simulink model "assignment1_c"  (R2021a)
settings: Solver=VariableStepAuto  StartTime=0.0  StopTime=10.0  RelTol=1e-3
undefined symbols (not defined in the file): c1, c2, k1, k2, m1, m2
settings Model: Creator=mluser  LastModifiedBy=mluser

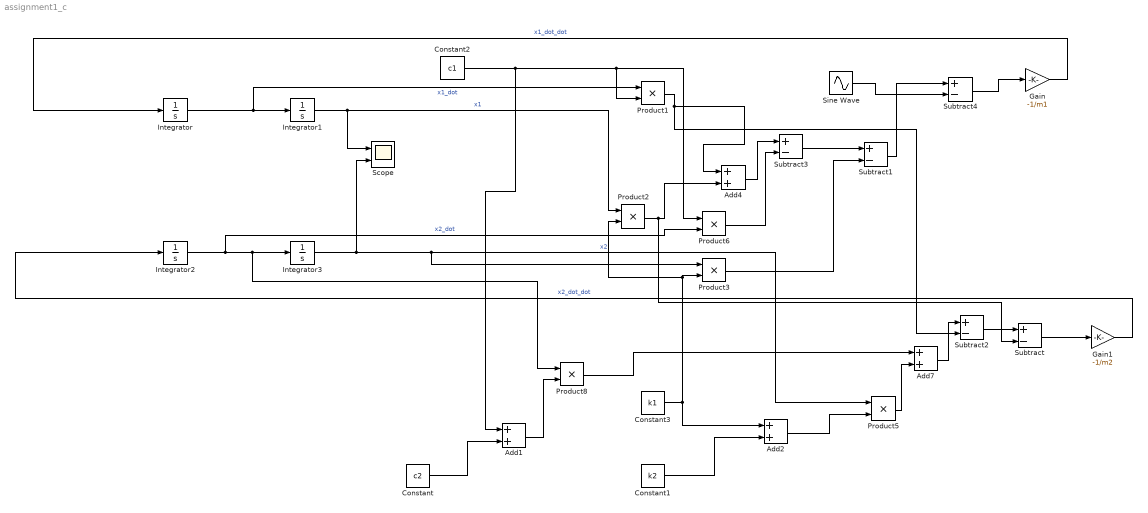
== system assignment1_c ==
  Add{1..2,4,7} (4 alike) : Sum
  Constant : Constant  Value=c2
  Constant1 : Constant  Value=k2
  Constant2 : Constant  Value=c1
  Constant3 : Constant  Value=k1
  Gain : Gain  Gain=-1/m1
  Gain1 : Gain  Gain=-1/m2
  Integrator{,1..3} (4 alike) : Integrator
  Product{1..3,5..6,8} (6 alike) : Product
  Scope : Scope  NumInputPorts=2
  Sine Wave : Sin  Amplitude=3  Frequency=10  SampleTime=0
  Subtract{,1..4} (5 alike) : Sum  Inputs=+-
  wires:
  Constant/1 -> Add1/2
  Product5/1 -> Add7/2
  Constant3/1 -> Product3/2, Product2/2, Add2/1
  Subtract3/1 -> Subtract1/1
  Product2/1 -> Subtract/2, Add4/2
  Constant2/1 -> Add1/1, Product6/1, Product1/2
  Gain1/1 -> Integrator2/1  "x2_dot_dot"
  Product8/1 -> Add7/1
  Sine Wave/1 -> Subtract4/2
  Add2/1 -> Product5/2
  Product1/1 -> Add4/1, Subtract2/2
  Integrator1/1 -> Scope/1, Product2/1  "x1"
  Product6/1 -> Subtract3/2
  Add1/1 -> Product8/2
  Subtract/1 -> Gain1/1
  Subtract2/1 -> Subtract/1
  Product3/1 -> Subtract1/2
  Constant1/1 -> Add2/2
  Integrator3/1 -> Scope/2, Product5/1, Product3/1  "x2"
  Subtract1/1 -> Subtract4/1
  Gain/1 -> Integrator/1  "x1_dot_dot"
  Add4/1 -> Subtract3/1
  Add7/1 -> Subtract2/1
  Subtract4/1 -> Gain/1
  Integrator/1 -> Product1/1, Integrator1/1  "x1_dot"
  Integrator2/1 -> Product6/2, Product8/1, Integrator3/1  "x2_dot"
